simulink model "MotorXploer"  (R2024b)
settings: Solver=FixedStepAuto  StartTime=0.0  StopTime=inf  FixedStep=0.001  RelTol=1e-3  EnableMultiTasking=on
undefined symbols (not defined in the file): Blocking, LF, Non
libraries: hdlsllib x5, amg_usbconverter_n_connect_lib x3, cstblocks x1, simulink x1, waijung_addon_module x1
(part 2 of 2)

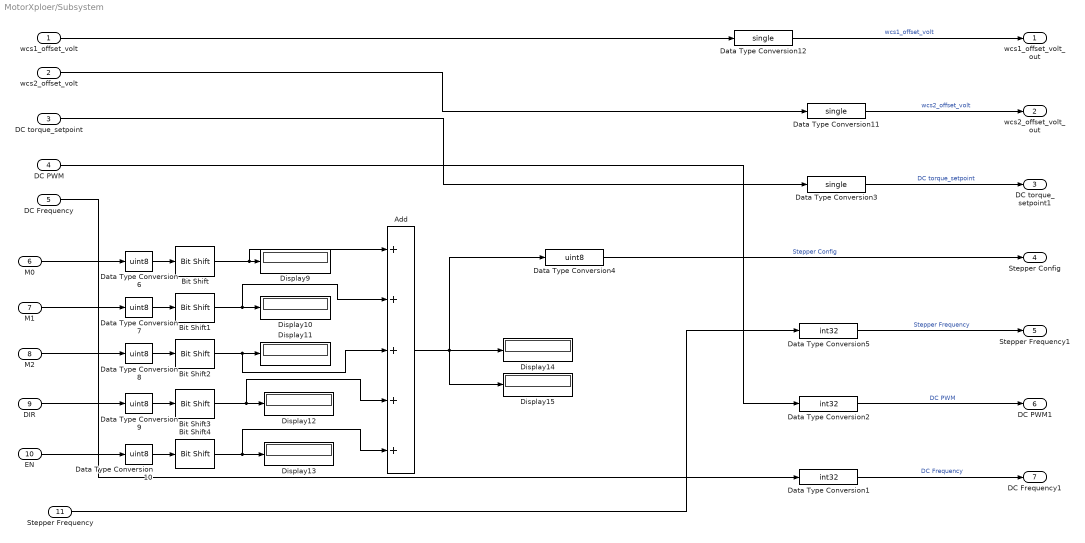
== system MotorXploer/Subsystem ==
  wcs1_offset_volt : Inport
  wcs2_offset_volt : Inport  Port=2
  DC torque_setpoint : Inport  Port=3
  DC PWM : Inport  Port=4
  DC Frequency : Inport  Port=5
  M0 : Inport  Port=6
  M1 : Inport  Port=7
  M2 : Inport  Port=8
  DIR : Inport  Port=9
  EN : Inport  Port=10
  Stepper Frequency : Inport  Port=11
  Add : Sum  Inputs=+++++
  Bit Shift : hdlsllib/Logic and Bit Operations/Bit Shift  mode=Shift Left Logical  N=4
  Bit Shift1 : hdlsllib/Logic and Bit Operations/Bit Shift  mode=Shift Left Logical  N=3
  Bit Shift2 : hdlsllib/Logic and Bit Operations/Bit Shift  mode=Shift Left Logical  N=2
  Bit Shift3 : hdlsllib/Logic and Bit Operations/Bit Shift  mode=Shift Left Logical  N=1
  Bit Shift4 : hdlsllib/Logic and Bit Operations/Bit Shift  mode=Shift Left Logical  N=0
  Data Type Conversion1 : DataTypeConversion  OutDataTypeStr=int32  SaturateOnIntegerOverflow=off  RndMeth=Floor
  Data Type Conversion{4,6..10} (6 alike) : DataTypeConversion  OutDataTypeStr=uint8  SaturateOnIntegerOverflow=off  RndMeth=Floor
  Data Type Conversion11 : DataTypeConversion  OutDataTypeStr=single  SaturateOnIntegerOverflow=off  RndMeth=Floor
  Data Type Conversion12 : DataTypeConversion  OutDataTypeStr=single  SaturateOnIntegerOverflow=off  RndMeth=Floor
  Data Type Conversion2 : DataTypeConversion  OutDataTypeStr=int32  SaturateOnIntegerOverflow=off  RndMeth=Floor
  Data Type Conversion3 : DataTypeConversion  OutDataTypeStr=single  SaturateOnIntegerOverflow=off  RndMeth=Floor
  Data Type Conversion5 : DataTypeConversion  OutDataTypeStr=int32  SaturateOnIntegerOverflow=off  RndMeth=Floor
  Display{9..15} (7 alike) : Display
      Display10 settings: Format=binary (Stored Integer)
      Display11 settings: Format=binary (Stored Integer)
      Display12 settings: Format=binary (Stored Integer)
      Display13 settings: Format=binary (Stored Integer)
      Display14 settings: Format=binary (Stored Integer)
      Display9 settings: Format=binary (Stored Integer)
  wcs1_offset_volt_out : Outport
  wcs2_offset_volt_out : Outport  Port=2
  DC torque_setpoint1 : Outport  Port=3
  Stepper Config : Outport  Port=4
  Stepper Frequency1 : Outport  Port=5
  DC PWM1 : Outport  Port=6
  DC Frequency1 : Outport  Port=7
  wires:
  Bit Shift/1 -> Display9/1, Add/1
  Data Type Conversion8/1 -> Bit Shift2/1
  EN/1 -> Data Type Conversion10/1
  Data Type Conversion6/1 -> Bit Shift/1
  DC torque_setpoint/1 -> Data Type Conversion3/1
  Data Type Conversion2/1 -> DC PWM1/1  "DC PWM"
  Data Type Conversion7/1 -> Bit Shift1/1
  Data Type Conversion10/1 -> Bit Shift4/1
  DC PWM/1 -> Data Type Conversion2/1
  Bit Shift3/1 -> Display12/1, Add/4
  Data Type Conversion12/1 -> wcs1_offset_volt_out/1  "wcs1_offset_volt"
  Add/1 -> Display15/1, Display14/1, Data Type Conversion4/1
  Bit Shift2/1 -> Display11/1, Add/3
  Stepper Frequency/1 -> Data Type Conversion5/1
  M1/1 -> Data Type Conversion7/1
  Bit Shift1/1 -> Display10/1, Add/2
  Bit Shift4/1 -> Display13/1, Add/5
  M0/1 -> Data Type Conversion6/1
  Data Type Conversion9/1 -> Bit Shift3/1
  Data Type Conversion11/1 -> wcs2_offset_volt_out/1  "wcs2_offset_volt"
  M2/1 -> Data Type Conversion8/1
  wcs1_offset_volt/1 -> Data Type Conversion12/1
  DC Frequency/1 -> Data Type Conversion1/1
  wcs2_offset_volt/1 -> Data Type Conversion11/1
  Data Type Conversion1/1 -> DC Frequency1/1  "DC Frequency"
  DIR/1 -> Data Type Conversion9/1
  Data Type Conversion4/1 -> Stepper Config/1  "Stepper Config"
  Data Type Conversion3/1 -> DC torque_setpoint1/1  "DC torque_setpoint"
  Data Type Conversion5/1 -> Stepper Frequency1/1  "Stepper Frequency"

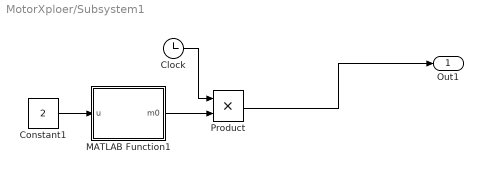
== system MotorXploer/Subsystem1 ==
  Clock : Clock
  Constant1 : Constant  Value=2
  MATLAB Function1 : MATLAB Function  TreatAsAtomicUnit=on
  Product : Product
  Out1 : Outport
  wires:
  Clock/1 -> Product/1
  Constant1/1 -> MATLAB Function1/1(u)
  MATLAB Function1/1(m0) -> Product/2
  Product/1 -> Out1/1

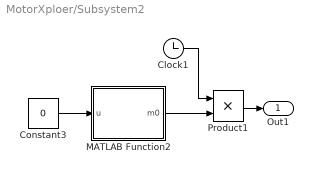
== system MotorXploer/Subsystem2 ==
  Clock1 : Clock
  Constant3 : Constant  Value=0
  MATLAB Function2 : MATLAB Function  TreatAsAtomicUnit=on
  Product1 : Product
  Out1 : Outport
  wires:
  MATLAB Function2/1(m0) -> Product1/2
  Constant3/1 -> MATLAB Function2/1(u)
  Clock1/1 -> Product1/1
  Product1/1 -> Out1/1

== matlab function MotorXploer/Subsystem1/MATLAB Function1 ==
  data: u input; m0 output
function m0  = fcn(u)
    % Initialize outputs
    m0 = 0;
    % Determine outputs based on input u
    if u == 0
        m0 = 0;
    elseif u == 1
        m0 = 1;
    elseif u == 2
        m0 = 10;
    elseif u == 3
        m0 = 50;
    elseif u == 4
        m0 = 100;
    elseif u == 5
        m0 = 500;
    elseif u == 6
        m0 = 1000;
    elseif u == 7
        m0 = 5000;
        elseif u == 8
        m0 = 10000;
        elseif u == 9
        m0 = 20000;
        elseif u == 10
        m0 = 50000;
        elseif u == 11
        m0 = 75000;
        elseif u == 12
        m0 = 100000;
    else
        % Handle invalid input
        error('Input u must be an integer between 0 and 7');
    end
end

== matlab function MotorXploer/MATLAB Function ==
  data: u input; m0 output; m1 output; m2 output
function [m0, m1, m2] = fcn(u)
    % Initialize outputs
    m0 = 0;
    m1 = 0;
    m2 = 0;
    
    % Determine outputs based on input u
    if u == 0
        m0 = 0; m1 = 0; m2 = 0;
    elseif u == 1
        m0 = 1; m1 = 0; m2 = 0;
    elseif u == 2
        m0 = 0; m1 = 1; m2 = 0;
    elseif u == 3
        m0 = 1; m1 = 1; m2 = 0;
    elseif u == 4
        m0 = 0; m1 = 0; m2 = 1;
    elseif u == 5
        m0 = 1; m1 = 0; m2 = 1;
    elseif u == 6
        m0 = 0; m1 = 1; m2 = 1;
    elseif u == 7
        m0 = 1; m1 = 1; m2 = 1;
    else
        % Handle invalid input
        error('Input u must be an integer between 0 and 7');
    end
end

== matlab function MotorXploer/Subsystem2/MATLAB Function2 ==
  data: u input; m0 output
function m0  = fcn(u)
    % Initialize outputs
    m0 = 0;
    % Determine outputs based on input u
    if u == 0
        m0 = 0;
    elseif u == 1
        m0 = 0.0001;
    elseif u == 2
        m0 = 0.0005;
    elseif u == 3
        m0 = 0.001;
    elseif u == 4
        m0 = 0.005;
    elseif u == 5
        m0 = 0.0075;
    elseif u == 6
        m0 = 0.01;
    elseif u == 7
        m0 = 0.025;
        elseif u == 8
        m0 = 0.05;
        elseif u == 9
        m0 = 0.075;
        elseif u == 10
        m0 = 0.1;
        elseif u == 11
        m0 = 0.5;
        elseif u == 12
        m0 = 1;
    else
        % Handle invalid input
        error('Input u must be an integer between 0 and 7');
    end
end

== matlab function MotorXploer/Loss Detector ==
  settings: updateMethod=DISCRETE
  data: frequency input; step_loss_detected output; angular_velocity input; elapsed_time input; lost_steps output; position_error output; steps_per_rev input; expected_step output
function [step_loss_detected, lost_steps, position_error, expected_step] = detect_loss(frequency, angular_velocity, elapsed_time, steps_per_rev)
% Inputs:
% frequency: Drive frequency of the motor (Hz)
% angular_velocity: Measured angular velocity (rad/s)
% elapsed_time: Time since the start (s)
% steps_per_rev: Number of steps per revolution of the motor (integer)

% Outputs:
% step_loss_detected: Boolean (1 if step loss is detected, 0 otherwise)
% lost_steps: Total accumulated lost steps
% position_error: Difference between commanded and actual position (radians)
% expected_step: Commanded step count based on drive frequency

    % Define persistent variables
    persistent accumulated_lost_steps prev_elapsed_time total_expected_steps;
    if isempty(accumulated_lost_steps)
        accumulated_lost_steps = 0; % Initialize lost steps
        prev_elapsed_time = 0; % Initialize previous elapsed time
        total_expected_steps = 0; % Initialize total expected steps
    end

    % Calculate step angle
    step_angle = 2 * pi / steps_per_rev;

    % Calculate time increment
    time_increment = elapsed_time - prev_elapsed_time;

    % Update previous elapsed time
    prev_elapsed_time = elapsed_time;

    % Calculate commanded steps incrementally
    commanded_steps_increment = frequency * time_increment;

    % Update total expected steps
    total_expected_steps = total_expected_steps + commanded_steps_increment;

    % Convert total expected steps to an integer
    expected_step = (total_expected_steps);

    % Commanded position in radians
    commanded_position = total_expected_steps * step_angle;


    % Actual position in radians based on angular velocity
    actual_position = angular_velocity * elapsed_time;

    % Position error
    position_error = commanded_position - actual_position;

    % Calculate incremental lost steps for this cycle
    incremental_lost_steps = round(position_error / step_angle);

    % Update the persistent variable for cumulative lost steps
    accumulated_lost_steps = accumulated_lost_steps + incremental_lost_steps;

    % Assign cumulative lost steps to the output
    lost_steps = accumulated_lost_steps;

    % Detect step loss
    if abs(position_error) > (0.5 * step_angle)
        step_loss_detected = 1; % Step loss detected
    else
        step_loss_detected = 0; % No step loss
    end
end
